simulink model "model"  (R2023b)
settings: Solver=VariableStepAuto  StartTime=0.0  StopTime=5  FixedStep=Tsi/10  RelTol=1e-4
undefined symbols (not defined in the file): B, B0, DiscIntNeverNeededParam, grtot, Hpp, Imax, In, Jm, Kdp_si, Ke, Ki_si, Kip_si, Kp_si, Kpp_si, Kppph_si, Kpppl_si, Kt, Kv, L, max_ppa_si, max_ppv_si, R, tauGp, Umax
libraries: simulink x10, slctrl_linear x1
(part 1 of 2)
settings Model: Creator=Giulio  LastModifiedBy=nicol
settings OptimizationCC: ReuseModelBlockBuffer=off
settings DebuggingCC: UnconnectedInputMsg=warning  UnconnectedOutputMsg=warning  UnconnectedLineMsg=warning
settings ModelReferenceCC: EnableRefExpFcnMdlSchedulingChecks=on

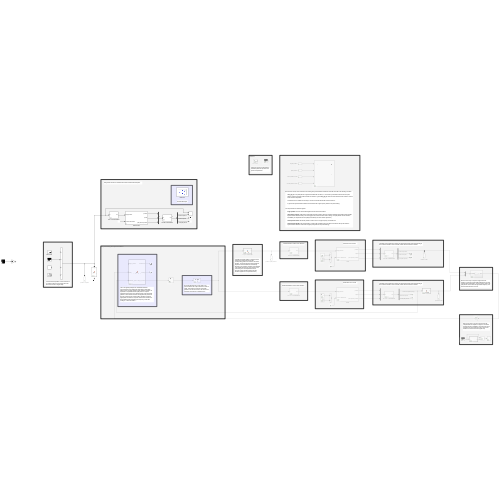
[thumbnail: Simulink's stored preview of the top-level diagram]
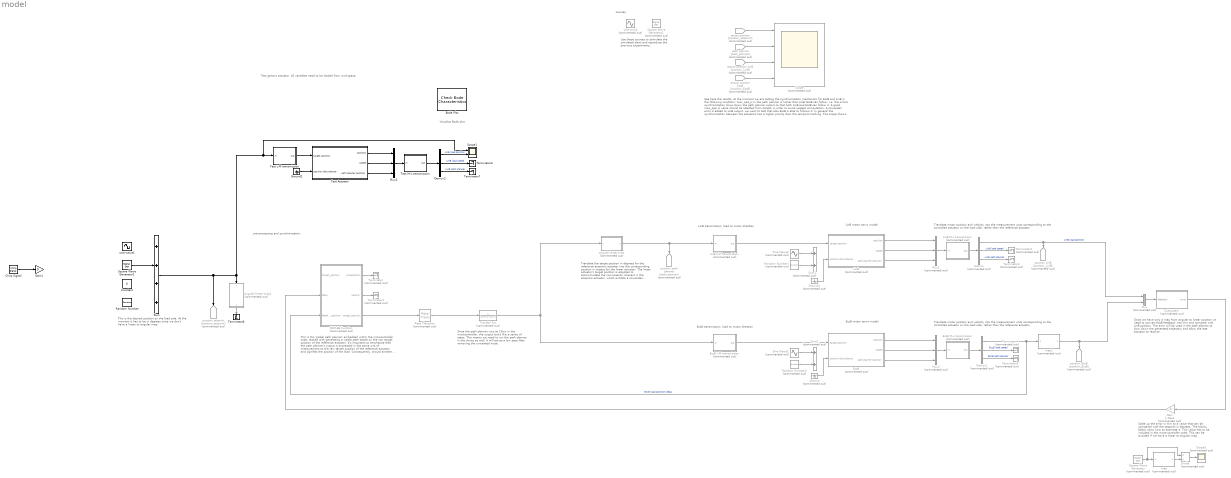
== system model ==
  note: This is the desired position on the load side. At the moment it has to be in degrees since we don't have a linear to angular map.
  note: This is the 'global path planner' embedded within the microcontroller code, tasked with generating a viable path based on the raw target position of the reference actuator. It's important to emphasize that the path planner's output is expressed in the same unit of measurement as the raw target position of the reference actuator and signifies the position of the load. Consequently, should another actuator be utilized, appropriate conversion is required. Note that the resolution of the generated path is limited by the frequency of the task running it, in this case 100Hz.
  note: sources
  note: Use these sources to stimulate the simulated plant and reproduce the previous experiments.
  note: pre-processing and synchronization
  note: Translate the target position in degrees for the reference eccentric actuator into the corresponding position in meters for the linear actuator. The linear actuator's target position is adjusted to accommodate the non-linearity inherent in the eccentric actuator, which exhibits a sinusoidal behavior due to the presence of a connecting rod. This adjustment ensures accurate synchronization between the two actuators (apart from unexpected blocks).
  note: Since the path planner runs at 10ms in the microcontroller, the output looks like a series of steps. This means we need to run the path planner in the drives as well. It will act as a low pass filter removing the unwanted noise.
  note: Translate motor position and velocity into the measurement units corresponding to the controlled actuator on the load side, rather than the reference actuator.
  note: Scale up the error in mm to a value that can be compared with the setpoint in degrees. The blocks below show how to estimate it. This value has to be included in the micro-controller code. This can be avoided if we have a linear to angular map.
  note: See here the results, at the moment we are testing the synchronization mechanism for EccB and LinB in the following condition:
      |
      | max_ppa_si in the path planner is higher that what EccB can follow, i.e. the online synchronization slows down the path planner output so that both LinB and EccB can follow it. A good max_ppa_si value should be selected from scratch in order to avoid useless computation.
      |
      | A sinusoidal error is added to LinB output, we want to test that also EccB is able to followo it.
      |
      | In general the synchronization between the actuators has a higher priority than the set-point tracking.
      |
      | The scope shows four different signals:
      |
      | target position : the raw commanded target that both drives should follow
      |
      | path planner position : path planner with double objective function (steer the actuators towards target position and maintain synchronization between them), note in the graph how, when the drives start to diverge, the path planner inverts direction immediately to compensate for thet (always bounded by the slow actuator dynamics).
      |
      | actual position LinB : LinB actual position to which we sum a high frequency sinusoidal error.
      |
      | actual position EccB : EccB actual position, it limits LinB acceleration at at the same time follows LinB (in this case the synchronization between motors has a higher priority than the set-point tracking).
  note: Since we have only a map from angular to linear position ve need to convert EccB feedback into mm and compare with LinB position. The error will be used in the path planner to slow down the generated trajectory and allow the late actuator to recover.
  note: LinB motor servo model
  note: EccB motor servo model
  note: LinB transmission: load to motor direction
  note: Translate motor position and velocity into the measurement units corresponding to the controlled actuator on the load side, rather than the reference actuator.
  note: EccB transmission: load to motor direction
  note: Visualize Bode plot
  note: Test generic actuator. All variables need to be loaded from workspace.
  Bode Plot : slctrl_linear/Check Bode  Characteristics  InstantiateOnLoad=on  SaveOperatingPoints=off  LinearizationIOs={'/Sum', 1, 'in', 'off', '';'/Demux2', 1, 'out', 'on', ''}  LinearizeAt=SnapshotTimes  SnapshotTimes=[0]  TriggerType=rising  SampleTime=auto  RateConversionMethod=zoh  PreWarpFreq=10  UseExactDelayModel=off  UseFullBlockNameLabels=off  UseBusSignalLabels=off  enabled=on  stopWhenAssertionFail=off  export=off  ViewDlgPos=[10 170 1856 825]  OpenViewOnLoad=off  LaunchViewOnOpen=on  FrequencyUnits=rad/s  MagnitudeUnits=dB  PhaseUnits=deg  TimeUnits=seconds  EnableUpperBound=off  UpperBoundFrequencies=[]  UpperBoundMagnitudes=[]  EnableLowerBound=off  LowerBoundFrequencies=[]  LowerBoundMagnitudes=[]
      settings: LibrarySourceBlock=slctrlblks/Linear Analysis Plots/Bode Plot  SaveToWorkspace=on  SaveName=sys
  Chirp Signal : simulink/Sources/Chirp Signal  f1=0.1  T=40  f2=5
  Constant : Constant  Value=0
  Demux : Demux  Commented=on  Outputs=3
  Demux1 : Demux  Commented=on  Outputs=3
  Demux2 : Demux  Outputs=3
  Divide : Product  Commented=on  Inputs=*/
  EccB : Subsystem  Commented=on  mask(Motor servo){Tsi=4e-5, Tsp=4e-4, Tspp=4e-4}
      mask DialogControl SamplingTimes Prompt: Sampling times
  EccB L-M transmission : Subsystem  Commented=on  mask(Transmission){gr_tot=2*pi*24.77/48, Direction=LOAD_TO_MOTOR}
      mask prompts: gr_tot "Total gear ratio"
      mask help: The total gear ratio represents the movement on motor side (in rad) correspondent to a displacement of one degree on load side.
      mask TypeOptions Direction: MOTOR_TO_LOAD | LOAD_TO_MOTOR
  EccB M-L transmission : Subsystem  Commented=on  mask(Transmission){gr_tot=2*pi*24.77/48, Direction=MOTOR_TO_LOAD}
      mask prompts: gr_tot "Total gear ratio"
      mask help: The total gear ratio represents the movement on motor side (in rad) correspondent to a displacement of one degree on load side.
      mask TypeOptions Direction: MOTOR_TO_LOAD | LOAD_TO_MOTOR
  Gain : Gain  Commented=on  Gain=1.48e4
  Gain1 : Gain  Gain=5
  Ground : Ground  Commented=on
  Ground1 : Ground  Commented=on
  Ground2 : Ground
  LinB : Subsystem  Commented=on  mask(Motor servo){Tsi=4e-5, Tsp=4e-4, Tspp=4e-4}
      mask DialogControl SamplingTimes Prompt: Sampling times
  LinB L-M transmission : Subsystem  Commented=on  mask(Transmission){gr_tot=1000*2*pi*174.72/48, Direction=LOAD_TO_MOTOR}
      mask prompts: gr_tot "Total gear ratio"
      mask help: The total gear ratio represents the movement on motor side (in rad) correspondent to a displacement of one meter on load side.
      mask TypeOptions Direction: MOTOR_TO_LOAD | LOAD_TO_MOTOR
  LinB M-L transmission : Subsystem  Commented=on  mask(Transmission){gr_tot=1000*2*pi*174.72/48, Direction=MOTOR_TO_LOAD}
      mask prompts: gr_tot "Total gear ratio"
      mask help: The total gear ratio represents the movement on motor side (in rad) correspondent to a displacement of one meter on load side.
      mask TypeOptions Direction: MOTOR_TO_LOAD | LOAD_TO_MOTOR
  MATLAB Function : MATLAB Function  Commented=on  TreatAsAtomicUnit=on  SystemSampleTime=Tspp  mask(High level path planner){Tspp=0.01, velocity_offset=1, Kppph_si=32.2971, Kpppl_si=3.2297, Hpp=12.5000, synch_to_target_ratio=1, max_ppv_si=155.6722, max_ppa_si=3.2297e+03}
      mask prompts: velocity_offset "Velocity hysteresis offset"; Kppph_si "Gain high limit"; Kpppl_si "Gain low limit"; Hpp "Exponential decay"; synch_to_target_ratio "Synch to target ratio"; max_ppv_si "Max velocity"; max_ppa_si "Max acceleration"
      mask help: Given a raw target trajectory, create a trajectory that all actuators are able to follow smoothly.
  Mux : Mux  Commented=on  Inputs=2
  Mux1 : Mux  Commented=on  Inputs=3
  Mux2 : Mux  Commented=on  Inputs=3
  Mux3 : Mux  Inputs=3
  Random Number : RandomNumber  Variance=1e-9  SampleTime=1e-3
  Random Number1 : RandomNumber  Commented=on  Variance=1e-6  SampleTime=1e-3
  Random Number2 : RandomNumber  Commented=on  Variance=1e-6  SampleTime=1e-3
  Rate Transition : RateTransition  Commented=on
  Scope : Scope  Commented=on  NumInputPorts=4
  Scope1 : Scope  NumInputPorts=2
  Scope3 : Scope  Commented=on
  Sine Wave1 : Sin  Commented=on  Amplitude=2e-4  Frequency=2*2*pi  SampleTime=0
  Sine Wave2 : Sin  Commented=on  Amplitude=2e-4  Frequency=2*2*pi  SampleTime=0
  Square Wave Generator : SignalGenerator  Commented=on  WaveForm=square
  Square Wave Generator1 : SignalGenerator  Commented=on  WaveForm=square  Amplitude=68.5  Frequency=0.5
  Square Wave Generator2 : SignalGenerator  WaveForm=square  Amplitude=-5  Frequency=0.4
  Subsystem : Subsystem  Commented=on
  Sum : Sum  Inputs=++++
  Sum1 : Sum  Commented=on
  Sum2 : Sum  Commented=on
  Terminator{,1..5} (6 alike) : Terminator  Commented=on
  Terminator6 : Terminator
  Terminator7 : Terminator
  Terminator8 : Terminator
  Test Actuator : Subsystem  mask(Motor servo){Tsi=4e-5, Tsp=4e-4, Tspp=4e-4}
      mask DialogControl SamplingTimes Prompt: Sampling times
  Test L-M transmission : Subsystem  mask(Transmission){gr_tot=grtot, Direction=LOAD_TO_MOTOR}
      mask prompts: gr_tot "Total gear ratio"
      mask help: The total gear ratio represents the movement on motor side (in rad) correspondent to a displacement of one meter on load side.
      mask TypeOptions Direction: MOTOR_TO_LOAD | LOAD_TO_MOTOR
  Test M-L transmission : Subsystem  mask(Transmission){gr_tot=grtot, Direction=MOTOR_TO_LOAD}
      mask prompts: gr_tot "Total gear ratio"
      mask help: The total gear ratio represents the movement on motor side (in rad) correspondent to a displacement of one meter on load side.
      mask TypeOptions Direction: MOTOR_TO_LOAD | LOAD_TO_MOTOR
  Transfer Fcn : TransferFcn  Commented=on  Denominator=[1/(2*pi*10) 1]
  actual position EccB : From  Commented=on  GotoTag=position_EccB
  actual position LinB : From  Commented=on  GotoTag=position_LinB
  angular-linear-map : MATLAB Function  Commented=on  TreatAsAtomicUnit=on
  angular-linear-map2 : MATLAB Function  Commented=on  TreatAsAtomicUnit=on
  map : MATLAB Function  Commented=on  TreatAsAtomicUnit=on
  map1 : MATLAB Function  Commented=on  TreatAsAtomicUnit=on
  path planner : From  Commented=on  GotoTag=path_planner
  position EccB : Goto  Commented=on  GotoTag=position_EccB
  position LinB : Goto  Commented=on  GotoTag=position_LinB
  position path planner : Goto  Commented=on  GotoTag=path_planner
  position setpoint : Goto  Commented=on  GotoTag=position_setpoint
  sine-wave : Sin  Commented=on  Amplitude=2.5e-3  Frequency=2*pi*2  SampleTime=0
  sine-wave1 : Sin  Amplitude=2.5e-3  Frequency=2*pi*17*3  SampleTime=0
  target position : From  Commented=on  GotoTag=position_setpoint
  wires:
  MATLAB Function/1(acceleration) -> Terminator/1
  MATLAB Function/2(velocity) -> Terminator1/1
  LinB M-L transmission/1(out) -> Demux/1
  Mux1/1 -> LinB M-L transmission/1(in)
  LinB/2(speed) -> Mux1/2
  LinB/1(position) -> Mux1/1
  LinB L-M transmission/1(out) -> LinB/1(target position)
  LinB/3(path planner position) -> Mux1/3
  Demux/2 -> Terminator2/1  "LinB load speed"
  Demux/3 -> Terminator3/1  "LinB path planner"
  EccB L-M transmission/1(out) -> EccB/1(target position)
  EccB/1(position) -> Mux2/1
  EccB/2(speed) -> Mux2/2
  EccB/3(path planner position) -> Mux2/3
  Mux2/1 -> EccB M-L transmission/1(in)
  EccB M-L transmission/1(out) -> Demux1/1
  Demux1/1 -> map1/1("x "), MATLAB Function/3(feedback_position)  "EccB load position [deg]"
  Demux1/2 -> Terminator4/1  "EccB load speed"
  Demux1/3 -> Terminator5/1  "EccB path planner"
  Mux/1 -> Subsystem/1(feedback)
  Transfer Fcn/1 -> EccB L-M transmission/1(in), angular-linear-map/1("x ")
  angular-linear-map/1(x) -> LinB L-M transmission/1(in), position path planner/1
  Subsystem/1(error) -> Gain/1
  map/1(x) -> Divide/2
  Square Wave Generator/1 -> Divide/1, map/1("x ")
  Divide/1 -> Scope3/1
  Gain/1 -> MATLAB Function/2(delay)
  Demux/1 -> position LinB/1, Mux/1  "LinB load position"
  actual position EccB/1 -> Scope/4
  actual position LinB/1 -> Scope/3
  target position/1 -> Scope/1
  path planner/1 -> Scope/2
  MATLAB Function/3(target_position) -> Rate Transition/1
  Rate Transition/1 -> Transfer Fcn/1
  map1/1(x) -> Mux/2, position EccB/1
  Sine Wave1/1 -> Sum1/1
  Random Number2/1 -> Sum1/2
  Random Number1/1 -> Sum2/2
  Sine Wave2/1 -> Sum2/1
  Ground/1 -> EccB/2(position disturbance)
  Ground1/1 -> LinB/2(position disturbance)
  Test L-M transmission/1(out) -> Test Actuator/1(target position)
  Test Actuator/3(path planner position) -> Mux3/3
  Test Actuator/2(speed) -> Mux3/2
  Mux3/1 -> Test M-L transmission/1(in)
  Test Actuator/1(position) -> Mux3/1
  Ground2/1 -> Test Actuator/2(position disturbance)
  Demux2/2 -> Terminator6/1  "LinB load speed"
  Demux2/3 -> Terminator7/1  "LinB path planner"
  Test M-L transmission/1(out) -> Demux2/1
  Demux2/1 -> Scope1/2  "LinB load position"
  Sum/1 -> position setpoint/1, Scope1/1, Test L-M transmission/1(in), angular-linear-map2/1("x ")
  angular-linear-map2/1(x) -> Terminator8/1
  Chirp Signal/1 -> Gain1/1
  Square Wave Generator2/1 -> Sum/2

== system model/EccB ==
  note: position control loop
  note: Employ a rate transmission block featuring a unity delay to replicate the time disparity between the sampling intervals of the position and current controllers.
  note: The position regulator takes multiple inputs, including the position setpoint, position feedback, and optionally, velocity and acceleration feedforward components. It then calculates and produces the necessary current signal to control the plant. This regulatory mechanism is implemented using a straightforward PID control scheme, complete with current saturation (limited to the motor's nominal current) and anti-windup provisions.
  note: motor path planner
  note: Drive internal path planner. It acts as low pass filter considering the physical limitation of the motor.
  target position : Inport
  position disturbance : Inport  Port=2
  Ground : Ground
  Rate Transition : RateTransition
  Sum : Sum
  Terminator{2..3,5..6} (4 alike) : Terminator
  current loop : Subsystem
  path planner : Subsystem  TreatAsAtomicUnit=on  SystemSampleTime=Tspp  mask(Drive internal path planner){Active=off, max_ppa_si=5.2360e+03, max_ppv_si=672.9990, Kppph_si=52.3599, Kpppl_si=5.2360, Hpp=12.5000}
      mask prompts: max_ppa_si "Max acceleration"; max_ppv_si "Max speed"; Kppph_si "High gain"; Kpppl_si "Low gain"; Hpp "Exponential"
      mask DialogControl ParameterGroupVar Prompt: Status
      mask DialogControl Container3 Prompt: Saturation
      mask DialogControl Container4 Prompt: Controller
  position regulator : Subsystem  TreatAsAtomicUnit=on  SystemSampleTime=Tsp  mask(Position PID controller){In=6.1800, Imax=27, Kpp_si=6, Kip_si=150, Kdp_si=0.06, FF_w_si=0, FF_a_si=0}
      mask prompts: In "Nominal current"; Imax "Max current"; Kpp_si "Proportional gain"; Kip_si "Integral gain"; Kdp_si "Derivative gain"; FF_w_si "Velocity feed forward gain"; FF_a_si "Acceleration feed forward gain"
      mask DialogControl Saturation Prompt: Saturation
      mask DialogControl Controller Prompt: Controller
  position : Outport
  speed : Outport  Port=2
  path planner position : Outport  Port=3
  wires:
  position regulator/1(current) -> Rate Transition/1
  current loop/1(position) -> Sum/1, position regulator/4(position_feedback)
  Rate Transition/1 -> current loop/1(current demand)
  current loop/4(voltage) -> Terminator5/1
  current loop/3(current) -> Terminator6/1
  path planner/2(motor speed) -> Terminator3/1
  path planner/1(motor acceleration) -> Terminator2/1
  Ground/1 -> position regulator/2(velocity feed forward), position regulator/1(acceleration feed forward)
  target position/1 -> path planner/1(motor_position)
  Sum/1 -> position/1
  path planner/3(motor position) -> path planner position/1, position regulator/3(position)
  current loop/2(velocity) -> speed/1
  position disturbance/1 -> Sum/2

== system model/EccB L-M transmission ==
  in : Inport
  Constant1 : Constant  Value=Direction
  Constant2 : Constant
  Equal : RelationalOperator  Operator===  OutDataTypeStr=boolean  RndMeth=Simplest  InputSameDT=off
  Switch : Switch  Criteria=u2 > Threshold  SaturateOnIntegerOverflow=off  InputSameDT=off
  gear ratio (L-M) : Gain  Gain=gr_tot
  inverse gear ratio (M-L) : Gain  Gain=1/gr_tot
  out : Outport
  wires:
  in/1 -> gear ratio (L-M)/1, inverse gear ratio (M-L)/1
  inverse gear ratio (M-L)/1 -> Switch/1
  gear ratio (L-M)/1 -> Switch/3
  Switch/1 -> out/1
  Constant1/1 -> Equal/1
  Equal/1 -> Switch/2
  Constant2/1 -> Equal/2

== system model/EccB M-L transmission ==
  in : Inport
  Constant1 : Constant  Value=Direction
  Constant2 : Constant
  Equal : RelationalOperator  Operator===  OutDataTypeStr=boolean  RndMeth=Simplest  InputSameDT=off
  Switch : Switch  Criteria=u2 > Threshold  SaturateOnIntegerOverflow=off  InputSameDT=off
  gear ratio (L-M) : Gain  Gain=gr_tot
  inverse gear ratio (M-L) : Gain  Gain=1/gr_tot
  out : Outport
  wires:
  in/1 -> gear ratio (L-M)/1, inverse gear ratio (M-L)/1
  inverse gear ratio (M-L)/1 -> Switch/1
  gear ratio (L-M)/1 -> Switch/3
  Switch/1 -> out/1
  Constant1/1 -> Equal/1
  Equal/1 -> Switch/2
  Constant2/1 -> Equal/2

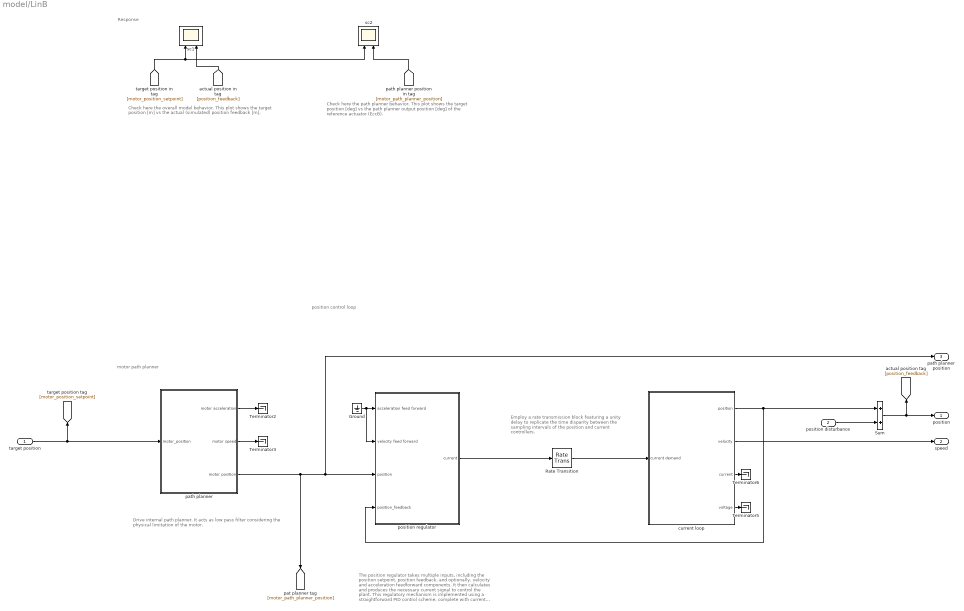
== system model/LinB ==
  note: position control loop
  note: Employ a rate transmission block featuring a unity delay to replicate the time disparity between the sampling intervals of the position and current controllers.
  note: The position regulator takes multiple inputs, including the position setpoint, position feedback, and optionally, velocity and acceleration feedforward components. It then calculates and produces the necessary current signal to control the plant. This regulatory mechanism is implemented using a straightforward PID control scheme, complete with current saturation (limited to the motor's nominal current) and anti-windup provisions.
  note: motor path planner
  note: Drive internal path planner. It acts as low pass filter considering the physical limitation of the motor.
  note: Response
  note: Check here the overall model behavior. This plot shows the target position [m] vs the actual (simulated) position feedback [m].
  note: Check here the path planner behavior. This plot shows the target position [deg] vs the path planner output position [deg] of the reference actuator (EccB).
  target position : Inport
  position disturbance : Inport  Port=2
  Ground : Ground
  Rate Transition : RateTransition
  Sum : Sum
  Terminator{2..3,5..6} (4 alike) : Terminator
  current loop : Subsystem
  path planner : Subsystem  TreatAsAtomicUnit=on  SystemSampleTime=Tspp  mask(Drive internal path planner){Active=off, max_ppa_si=2.0944e+03, max_ppv_si=656.2438, Kppph_si=20.9440, Kpppl_si=2.0944, Hpp=12.5000}
      mask prompts: max_ppa_si "Max acceleration"; max_ppv_si "Max speed"; Kppph_si "High gain"; Kpppl_si "Low gain"; Hpp "Exponential"
      mask DialogControl ParameterGroupVar Prompt: Status
      mask DialogControl Container3 Prompt: Saturation
      mask DialogControl Container4 Prompt: Controller
  position regulator : Subsystem  TreatAsAtomicUnit=on  SystemSampleTime=Tsp  mask(Position PID controller){In=4.2700, Imax=22, Kpp_si=2.5, Kip_si=50, Kdp_si=0.025, FF_w_si=0, FF_a_si=0}
      mask prompts: In "Nominal current"; Imax "Max current"; Kpp_si "Proportional gain"; Kip_si "Integral gain"; Kdp_si "Derivative gain"; FF_w_si "Velocity feed forward gain"; FF_a_si "Acceleration feed forward gain"
      mask DialogControl Saturation Prompt: Saturation
      mask DialogControl Controller Prompt: Controller
  sc1 : Scope  NumInputPorts=2
  sc2 : Scope  NumInputPorts=2
  position : Outport
  speed : Outport  Port=2
  path planner position : Outport  Port=3
  wires:
  path planner/3(motor position) -> path planner position/1, position regulator/3(position), [motor_path_planner_position]
  position regulator/1(current) -> Rate Transition/1
  current loop/1(position) -> Sum/1, position regulator/4(position_feedback)
  Rate Transition/1 -> current loop/1(current demand)
  current loop/4(voltage) -> Terminator5/1
  current loop/3(current) -> Terminator6/1
  path planner/2(motor speed) -> Terminator3/1
  path planner/1(motor acceleration) -> Terminator2/1
  Ground/1 -> position regulator/2(velocity feed forward), position regulator/1(acceleration feed forward)
  target position/1 -> [motor_position_setpoint], path planner/1(motor_position)
  current loop/2(velocity) -> speed/1
  [motor_position_setpoint] -> sc2/1, sc1/1
  [position_feedback] -> sc1/2
  [motor_path_planner_position] -> sc2/2
  position disturbance/1 -> Sum/2
  Sum/1 -> [position_feedback], position/1

== system model/LinB L-M transmission ==
  in : Inport
  Constant1 : Constant  Value=Direction
  Constant2 : Constant
  Equal : RelationalOperator  Operator===  OutDataTypeStr=boolean  RndMeth=Simplest  InputSameDT=off
  Switch : Switch  Criteria=u2 > Threshold  SaturateOnIntegerOverflow=off  InputSameDT=off
  gear ratio (L-M) : Gain  Gain=gr_tot
  inverse gear ratio (M-L) : Gain  Gain=1/gr_tot
  out : Outport
  wires:
  in/1 -> gear ratio (L-M)/1, inverse gear ratio (M-L)/1
  inverse gear ratio (M-L)/1 -> Switch/1
  gear ratio (L-M)/1 -> Switch/3
  Switch/1 -> out/1
  Constant1/1 -> Equal/1
  Equal/1 -> Switch/2
  Constant2/1 -> Equal/2

== system model/LinB M-L transmission ==
  in : Inport
  Constant1 : Constant  Value=Direction
  Constant2 : Constant
  Equal : RelationalOperator  Operator===  OutDataTypeStr=boolean  RndMeth=Simplest  InputSameDT=off
  Switch : Switch  Criteria=u2 > Threshold  SaturateOnIntegerOverflow=off  InputSameDT=off
  gear ratio (L-M) : Gain  Gain=gr_tot
  inverse gear ratio (M-L) : Gain  Gain=1/gr_tot
  out : Outport
  wires:
  in/1 -> gear ratio (L-M)/1, inverse gear ratio (M-L)/1
  inverse gear ratio (M-L)/1 -> Switch/1
  gear ratio (L-M)/1 -> Switch/3
  Switch/1 -> out/1
  Constant1/1 -> Equal/1
  Equal/1 -> Switch/2
  Constant2/1 -> Equal/2

== system model/Subsystem ==
  feedback : Inport
  MinMax : MinMax
  MinMax1 : MinMax  Function=max
  Selector : Selector  InputPortWidth=3  IndexOptions=Index vector (dialog)  Indices=1  OutputSizes=1
  Sum : Sum  Inputs=+-
  error : Outport
  wires:
  feedback/1 -> MinMax/1, MinMax1/1
  MinMax1/1 -> Sum/1
  MinMax/1 -> Sum/2
  Sum/1 -> Selector/1
  Selector/1 -> error/1

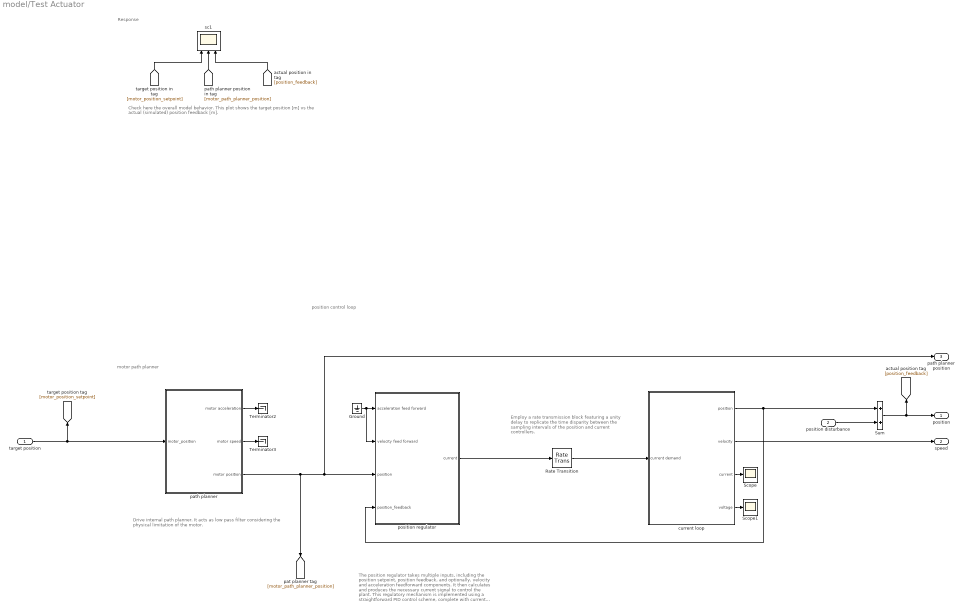
== system model/Test Actuator ==
  note: position control loop
  note: Employ a rate transmission block featuring a unity delay to replicate the time disparity between the sampling intervals of the position and current controllers.
  note: The position regulator takes multiple inputs, including the position setpoint, position feedback, and optionally, velocity and acceleration feedforward components. It then calculates and produces the necessary current signal to control the plant. This regulatory mechanism is implemented using a straightforward PID control scheme, complete with current saturation (limited to the motor's nominal current) and anti-windup provisions.
  note: motor path planner
  note: Drive internal path planner. It acts as low pass filter considering the physical limitation of the motor.
  note: Response
  note: Check here the overall model behavior. This plot shows the target position [m] vs the actual (simulated) position feedback [m].
  target position : Inport
  position disturbance : Inport  Port=2
  Ground : Ground
  Rate Transition : RateTransition
  Scope : Scope
  Scope1 : Scope
  Sum : Sum
  Terminator2 : Terminator
  Terminator3 : Terminator
  current loop : Subsystem
  path planner : Subsystem  TreatAsAtomicUnit=on  SystemSampleTime=Tspp  mask(Drive internal path planner){Active=off, max_ppa_si=max_ppa_si, max_ppv_si=max_ppv_si, Kppph_si=Kppph_si, Kpppl_si=Kpppl_si, Hpp=Hpp}
      mask prompts: max_ppa_si "Max acceleration"; max_ppv_si "Max speed"; Kppph_si "High gain"; Kpppl_si "Low gain"; Hpp "Exponential"
      mask DialogControl ParameterGroupVar Prompt: Status
      mask DialogControl Container3 Prompt: Saturation
      mask DialogControl Container4 Prompt: Controller
  position regulator : Subsystem  TreatAsAtomicUnit=on  SystemSampleTime=Tsp  mask(Position PID controller){In=In, Imax=Imax, Kpp_si=Kpp_si, Kip_si=Kip_si, Kdp_si=Kdp_si, FF_w_si=0, FF_a_si=0}
      mask prompts: In "Nominal current"; Imax "Max current"; Kpp_si "Proportional gain"; Kip_si "Integral gain"; Kdp_si "Derivative gain"; FF_w_si "Velocity feed forward gain"; FF_a_si "Acceleration feed forward gain"
      mask DialogControl Saturation Prompt: Saturation
      mask DialogControl Controller Prompt: Controller
  sc1 : Scope  NumInputPorts=3
  position : Outport
  speed : Outport  Port=2
  path planner position : Outport  Port=3
  wires:
  position regulator/1(current) -> Rate Transition/1
  current loop/1(position) -> Sum/1, position regulator/4(position_feedback)
  Rate Transition/1 -> current loop/1(current demand)
  current loop/4(voltage) -> Scope1/1
  current loop/3(current) -> Scope/1
  path planner/2(motor speed) -> Terminator3/1
  path planner/1(motor acceleration) -> Terminator2/1
  Ground/1 -> position regulator/2(velocity feed forward), position regulator/1(acceleration feed forward)
  target position/1 -> [motor_position_setpoint], path planner/1(motor_position)
  current loop/2(velocity) -> speed/1
  [motor_position_setpoint] -> sc1/1
  position disturbance/1 -> Sum/2
  Sum/1 -> [position_feedback], position/1
  [position_feedback] -> sc1/3
  [motor_path_planner_position] -> sc1/2
  path planner/3(motor position) -> [motor_path_planner_position], path planner position/1, position regulator/3(position)

== system model/Test L-M transmission ==
  in : Inport
  Constant1 : Constant  Value=Direction
  Constant2 : Constant
  Equal : RelationalOperator  Operator===  OutDataTypeStr=boolean  RndMeth=Simplest  InputSameDT=off
  Switch : Switch  Criteria=u2 > Threshold  SaturateOnIntegerOverflow=off  InputSameDT=off
  gear ratio (L-M) : Gain  Gain=gr_tot
  inverse gear ratio (M-L) : Gain  Gain=1/gr_tot
  out : Outport
  wires:
  in/1 -> gear ratio (L-M)/1, inverse gear ratio (M-L)/1
  inverse gear ratio (M-L)/1 -> Switch/1
  gear ratio (L-M)/1 -> Switch/3
  Switch/1 -> out/1
  Constant1/1 -> Equal/1
  Equal/1 -> Switch/2
  Constant2/1 -> Equal/2

== system model/Test M-L transmission ==
  in : Inport
  Constant1 : Constant  Value=Direction
  Constant2 : Constant
  Equal : RelationalOperator  Operator===  OutDataTypeStr=boolean  RndMeth=Simplest  InputSameDT=off
  Switch : Switch  Criteria=u2 > Threshold  SaturateOnIntegerOverflow=off  InputSameDT=off
  gear ratio (L-M) : Gain  Gain=gr_tot
  inverse gear ratio (M-L) : Gain  Gain=1/gr_tot
  out : Outport
  wires:
  in/1 -> gear ratio (L-M)/1, inverse gear ratio (M-L)/1
  inverse gear ratio (M-L)/1 -> Switch/1
  gear ratio (L-M)/1 -> Switch/3
  Switch/1 -> out/1
  Constant1/1 -> Equal/1
  Equal/1 -> Switch/2
  Constant2/1 -> Equal/2

== system model/EccB/current loop ==
  note: The current regulator receives input in the form of the desired current and current feedback from the plant, subsequently applying the requisite voltage to drive the BLDC motor. This regulation is achieved through the implementation of a PI controller, which incorporates voltage saturation (limited to the motor's nominal voltage) and anti-windup mechanisms.
  note: Second order BLDC motor model takes the desired voltage and the load inertia (adjusted for the motor side using the gear ratio) as inputs and produces outputs for position, velocity, and current. It serves as a basic representation solely for simulation purposes, with the potential for more detailed and improved implementation in future iterations.
  note: Here the Power supply could be modelled. Pay attention to this because on the car the voltage supply is not always constant and it has to be taken into account.
  note: First order BLDC motor model used to check that the parameter estimation is not to bad. Can be used as observer + Luenberg in the future if needed.
  current demand : Inport
  Scope : Scope  NumInputPorts=2
  Scope1 : Scope  NumInputPorts=2
  current regulator : Subsystem  TreatAsAtomicUnit=on  SystemSampleTime=Tsi  mask(Current PI controller){Umax=48, Un=36, Kp_si=0.9689, Ki_si=603.1858}
      mask prompts: Umax "Max voltage"; Un "Nominal voltage"; Kp_si "Proportional gain"; Ki_si "Integral gain"
      mask DialogControl Saturation Prompt: Saturation
      mask DialogControl Controller Prompt: Controller
  first order plant : Subsystem  mask(Motor first order plant){tauM=5.4400e-04, Kv=14.1372}
      mask prompts: tauM "Mechanical time constant"; Kv "Velocity constant"
      mask DialogControl Motor Prompt: Motor
  power supply : Subsystem
  second order plant : Subsystem  mask(Motor second order model){Ke=0.0706, R=0.16, L=2.5700e-04, Kt=0.0706, Jm=1.8290e-05, B=7.0915e-05, B0=0}
      mask prompts: Ke "Electrical constant"; R "Resistance"; L "Inductance"; Kt "Torque constant"; Jm "Motor inertia"; B "Viscous friction"; B0 "Static friction"
      mask DialogControl electrical Prompt: Electrical
      mask DialogControl Mechanical Prompt: Mechanical
  position : Outport
  velocity : Outport  Port=2
  current : Outport  Port=3
  voltage : Outport  Port=4
  wires:
  second order plant/2(velocity) -> Scope1/1, velocity/1
  current demand/1 -> current regulator/1(current)
  second order plant/1(position) -> Scope/1, position/1
  second order plant/3(current) -> current regulator/2(current_feedback), current/1
  power supply/1(voltage) -> second order plant/1(voltage), voltage/1
  current regulator/1(voltage) -> first order plant/1(voltage), power supply/1(voltage setpoint)
  first order plant/1(position) -> Scope/2
  first order plant/2(velocity) -> Scope1/2

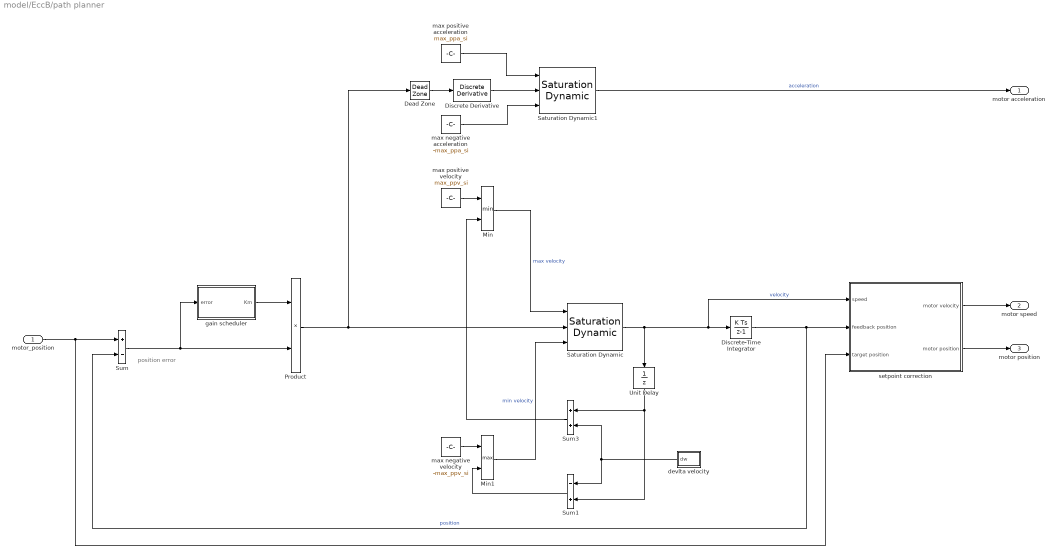
== system model/EccB/path planner ==
  note: position error
  motor_position : Inport
  Dead Zone : DeadZone  LowerValue=-0.01  UpperValue=0.01
  Discrete Derivative : simulink/Discrete/Discrete Derivative  gainval=1.0  ICPrevScaledInput=0.0  OutMin=[]  OutMax=[]  OutDataType=fixdt(1, 16)  OutScaling=2^-10  DoSatur=off
  Discrete-Time Integrator : DiscreteIntegrator  SampleTime=-1  ICPrevOutput=DiscIntNeverNeededParam  ICPrevScaledInput=DiscIntNeverNeededParam
  Min : MinMax  Inputs=2
  Min1 : MinMax  Function=max  Inputs=2
  Product : Product
  Saturation Dynamic : simulink/Discontinuities/Saturation Dynamic  OutMin=[]  OutMax=[]  OutDataTypeStr=Inherit: Same as second input  OutDataType=fixdt(1, 16)  OutScaling=2^-10  DoSatur=off
  Saturation Dynamic1 : simulink/Discontinuities/Saturation Dynamic  OutMin=[]  OutMax=[]  OutDataTypeStr=Inherit: Same as second input  OutDataType=fixdt(1, 16)  OutScaling=2^-10  DoSatur=off
  Sum : Sum  Inputs=+-
  Sum1 : Sum  Inputs=-+
  Sum3 : Sum
  Unit Delay : UnitDelay  SampleTime=-1  HasFrameUpgradeWarning=on
  devlta velocity : Subsystem
  gain scheduler : Subsystem
  max negative acceleration : Constant  Value=-max_ppa_si
  max negative velocity : Constant  Value=-max_ppv_si
  max positive acceleration : Constant  Value=max_ppa_si
  max positive velocity : Constant  Value=max_ppv_si
  setpoint correction : Subsystem
  motor acceleration : Outport
  motor speed : Outport  Port=2
  motor position : Outport  Port=3
  wires:
  Sum/1 -> gain scheduler/1(error), Product/2
  max positive velocity/1 -> Min/1
  Saturation Dynamic/1 -> setpoint correction/1(speed), Discrete-Time Integrator/1, Unit Delay/1  "velocity"
  devlta velocity/1(dw) -> Sum1/1, Sum3/2
  Sum3/1 -> Min/2
  max negative velocity/1 -> Min1/1
  Sum1/1 -> Min1/2
  Min1/1 -> Saturation Dynamic/3  "min velocity"
  Min/1 -> Saturation Dynamic/1  "max velocity"
  Discrete-Time Integrator/1 -> setpoint correction/2(feedback position), Sum/2  "position"
  Unit Delay/1 -> Sum1/2, Sum3/1
  max positive acceleration/1 -> Saturation Dynamic1/1
  max negative acceleration/1 -> Saturation Dynamic1/3
  Saturation Dynamic1/1 -> motor acceleration/1  "acceleration"
  Discrete Derivative/1 -> Saturation Dynamic1/2
  Dead Zone/1 -> Discrete Derivative/1
  setpoint correction/1(motor velocity) -> motor speed/1
  gain scheduler/1(Km) -> Product/1
  motor_position/1 -> setpoint correction/3(target position), Sum/1
  setpoint correction/2(motor position) -> motor position/1
  Product/1 -> Dead Zone/1, Saturation Dynamic/2

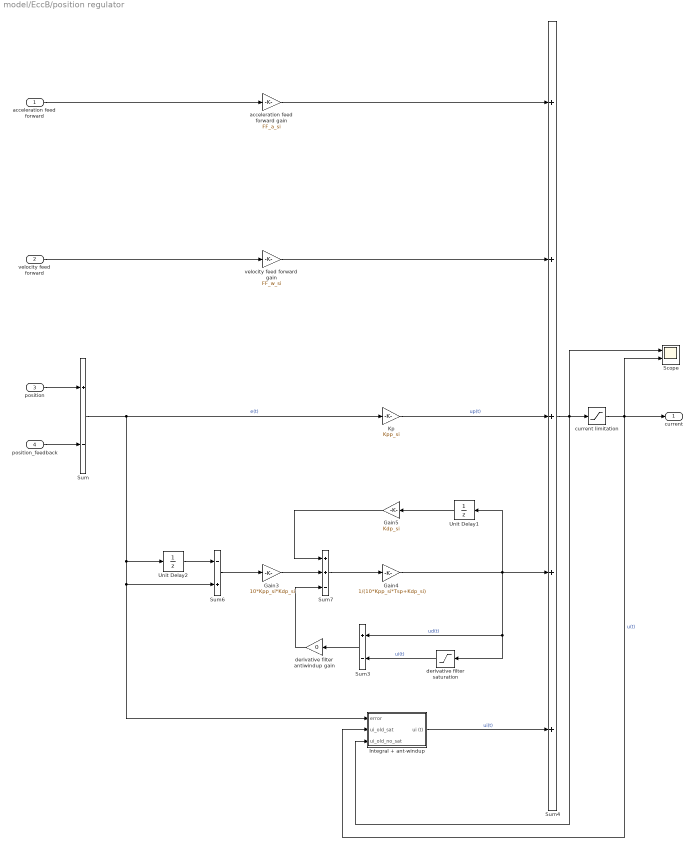
== system model/EccB/position regulator ==
  acceleration feed forward : Inport
  velocity feed forward : Inport  Port=2
  position : Inport  Port=3
  position_feedback : Inport  Port=4
  Gain3 : Gain  Gain=10*Kpp_si*Kdp_si
  Gain4 : Gain  Gain=1/(10*Kpp_si*Tsp+Kdp_si)
  Gain5 : Gain  Gain=Kdp_si
  Integral + ant-windup : Subsystem
  Kp : Gain  Gain=Kpp_si
  Scope : Scope  NumInputPorts=2
  Sum : Sum  Inputs=+-
  Sum3 : Sum  Inputs=+-
  Sum4 : Sum  Inputs=+++++
  Sum6 : Sum  Inputs=-+
  Sum7 : Sum  Inputs=++-
  Unit Delay1 : UnitDelay  SampleTime=-1  HasFrameUpgradeWarning=on
  Unit Delay2 : UnitDelay  SampleTime=-1  HasFrameUpgradeWarning=on
  acceleration feed forward gain : Gain  Gain=FF_a_si
  current limitation : Saturate  UpperLimit=Imax  LowerLimit=-Imax
  derivative filter antiwindup gain : Gain  Gain=0
  derivative filter saturation : Saturate  UpperLimit=Imax/2  LowerLimit=-Imax/2
  velocity feed forward gain : Gain  Gain=FF_w_si
  current : Outport
  wires:
  acceleration feed forward gain/1 -> Sum4/1
  acceleration feed forward/1 -> acceleration feed forward gain/1
  velocity feed forward gain/1 -> Sum4/2
  velocity feed forward/1 -> velocity feed forward gain/1
  Sum7/1 -> Gain4/1
  current limitation/1 -> current/1, Scope/2, Integral + ant-windup/2(ui_old_sat)  "u(t)"
  Unit Delay2/1 -> Sum6/1
  Sum6/1 -> Gain3/1
  Unit Delay1/1 -> Gain5/1
  Kp/1 -> Sum4/3  "up(t)"
  Sum/1 -> Kp/1, Integral + ant-windup/1(error), Sum6/2, Unit Delay2/1  "e(t)"
  Gain3/1 -> Sum7/2
  Gain5/1 -> Sum7/1
  Gain4/1 -> Sum4/4, derivative filter saturation/1, Sum3/1, Unit Delay1/1  "ud(t)"
  Sum3/1 -> derivative filter antiwindup gain/1
  derivative filter saturation/1 -> Sum3/2  "ui(t)"
  derivative filter antiwindup gain/1 -> Sum7/3
  Integral + ant-windup/1(ui (t)) -> Sum4/5  "ui(t)"
  Sum4/1 -> Scope/1, current limitation/1, Integral + ant-windup/3(ui_old_no_sat)
  position/1 -> Sum/1
  position_feedback/1 -> Sum/2

== system model/LinB/current loop ==
  note: The current regulator receives input in the form of the desired current and current feedback from the plant, subsequently applying the requisite voltage to drive the BLDC motor. This regulation is achieved through the implementation of a PI controller, which incorporates voltage saturation (limited to the motor's nominal voltage) and anti-windup mechanisms.
  note: Second order BLDC motor model takes the desired voltage and the load inertia (adjusted for the motor side using the gear ratio) as inputs and produces outputs for position, velocity, and current. It serves as a basic representation solely for simulation purposes, with the potential for more detailed and improved implementation in future iterations.
  note: Here the Power supply could be modelled. Pay attention to this because on the car the voltage supply is not always constant and it has to be taken into account.
  note: First order BLDC motor model used to check that the parameter estimation is not to bad. Can be used as observer + Luenberg in the future if needed.
  current demand : Inport
  Scope : Scope  NumInputPorts=2
  Scope1 : Scope  NumInputPorts=2
  current regulator : Subsystem  TreatAsAtomicUnit=on  SystemSampleTime=Tsi  mask(Current PI controller){Umax=48, Un=36, Kp_si=1.9302, Ki_si=1.9943e+03}
      mask prompts: Umax "Max voltage"; Un "Nominal voltage"; Kp_si "Proportional gain"; Ki_si "Integral gain"
      mask DialogControl Saturation Prompt: Saturation
      mask DialogControl Controller Prompt: Controller
  first order plant : Subsystem  mask(Motor first order plant){tauM=7.7800e-04, Kv=13.7183}
      mask prompts: tauM "Mechanical time constant"; Kv "Velocity constant"
      mask DialogControl Motor Prompt: Motor
  power supply : Subsystem
  second order plant : Subsystem  mask(Motor second order model){Ke=0.0728, R=0.5290, L=5.1200e-04, Kt=0.0728, Jm=9.2000e-06, B=3.6682e-05, B0=0}
      mask prompts: Ke "Electrical constant"; R "Resistance"; L "Inductance"; Kt "Torque constant"; Jm "Motor inertia"; B "Viscous friction"; B0 "Static friction"
      mask DialogControl electrical Prompt: Electrical
      mask DialogControl Mechanical Prompt: Mechanical
  position : Outport
  velocity : Outport  Port=2
  current : Outport  Port=3
  voltage : Outport  Port=4
  wires:
  second order plant/2(velocity) -> Scope1/1, velocity/1
  current demand/1 -> current regulator/1(current)
  second order plant/1(position) -> Scope/1, position/1
  second order plant/3(current) -> current regulator/2(current_feedback), current/1
  power supply/1(voltage) -> second order plant/1(voltage), voltage/1
  current regulator/1(voltage) -> first order plant/1(voltage), power supply/1(voltage setpoint)
  first order plant/1(position) -> Scope/2
  first order plant/2(velocity) -> Scope1/2

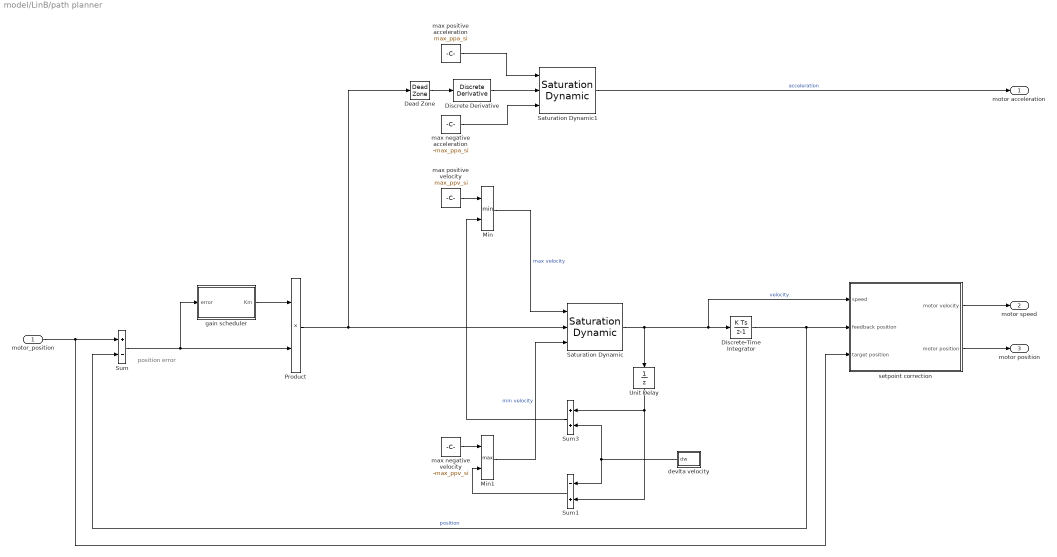
== system model/LinB/path planner ==
  note: position error
  motor_position : Inport
  Dead Zone : DeadZone  LowerValue=-0.01  UpperValue=0.01
  Discrete Derivative : simulink/Discrete/Discrete Derivative  gainval=1.0  ICPrevScaledInput=0.0  OutMin=[]  OutMax=[]  OutDataType=fixdt(1, 16)  OutScaling=2^-10  DoSatur=off
  Discrete-Time Integrator : DiscreteIntegrator  SampleTime=Tspp  ICPrevOutput=DiscIntNeverNeededParam  ICPrevScaledInput=DiscIntNeverNeededParam
  Min : MinMax  Inputs=2
  Min1 : MinMax  Function=max  Inputs=2
  Product : Product
  Saturation Dynamic : simulink/Discontinuities/Saturation Dynamic  OutMin=[]  OutMax=[]  OutDataTypeStr=Inherit: Same as second input  OutDataType=fixdt(1, 16)  OutScaling=2^-10  DoSatur=off
  Saturation Dynamic1 : simulink/Discontinuities/Saturation Dynamic  OutMin=[]  OutMax=[]  OutDataTypeStr=Inherit: Same as second input  OutDataType=fixdt(1, 16)  OutScaling=2^-10  DoSatur=off
  Sum : Sum  Inputs=+-
  Sum1 : Sum  Inputs=-+
  Sum3 : Sum
  Unit Delay : UnitDelay  SampleTime=-1  HasFrameUpgradeWarning=on
  devlta velocity : Subsystem
  gain scheduler : Subsystem
  max negative acceleration : Constant  Value=-max_ppa_si
  max negative velocity : Constant  Value=-max_ppv_si
  max positive acceleration : Constant  Value=max_ppa_si
  max positive velocity : Constant  Value=max_ppv_si
  setpoint correction : Subsystem
  motor acceleration : Outport
  motor speed : Outport  Port=2
  motor position : Outport  Port=3
  wires:
  Sum/1 -> gain scheduler/1(error), Product/2
  max positive velocity/1 -> Min/1
  Saturation Dynamic/1 -> setpoint correction/1(speed), Discrete-Time Integrator/1, Unit Delay/1  "velocity"
  devlta velocity/1(dw) -> Sum1/1, Sum3/2
  Sum3/1 -> Min/2
  max negative velocity/1 -> Min1/1
  Sum1/1 -> Min1/2
  Min1/1 -> Saturation Dynamic/3  "min velocity"
  Min/1 -> Saturation Dynamic/1  "max velocity"
  Discrete-Time Integrator/1 -> setpoint correction/2(feedback position), Sum/2  "position"
  Unit Delay/1 -> Sum1/2, Sum3/1
  max positive acceleration/1 -> Saturation Dynamic1/1
  max negative acceleration/1 -> Saturation Dynamic1/3
  Saturation Dynamic1/1 -> motor acceleration/1  "acceleration"
  Discrete Derivative/1 -> Saturation Dynamic1/2
  Dead Zone/1 -> Discrete Derivative/1
  setpoint correction/1(motor velocity) -> motor speed/1
  gain scheduler/1(Km) -> Product/1
  motor_position/1 -> setpoint correction/3(target position), Sum/1
  setpoint correction/2(motor position) -> motor position/1
  Product/1 -> Dead Zone/1, Saturation Dynamic/2

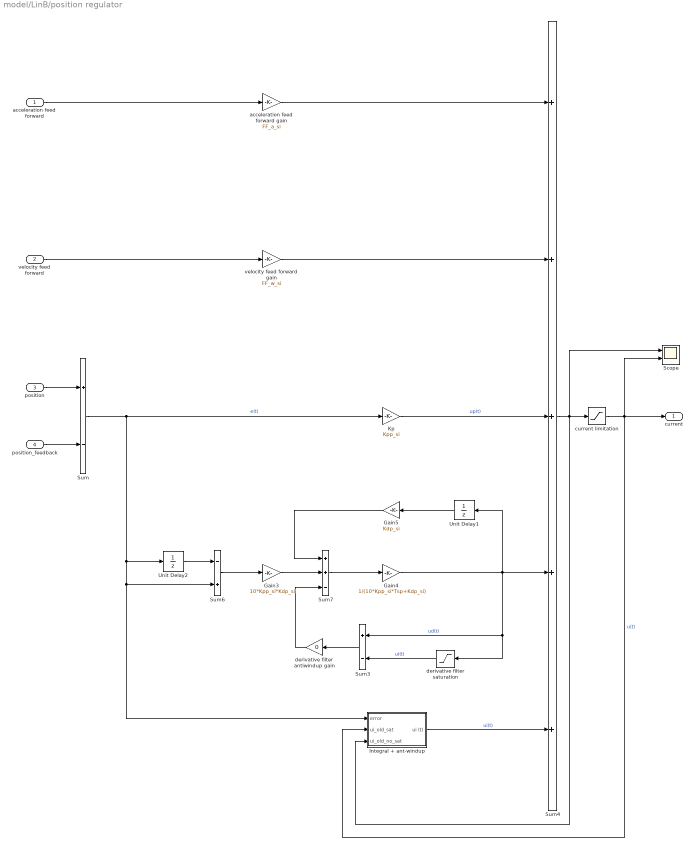
== system model/LinB/position regulator ==
  acceleration feed forward : Inport
  velocity feed forward : Inport  Port=2
  position : Inport  Port=3
  position_feedback : Inport  Port=4
  Gain3 : Gain  Gain=10*Kpp_si*Kdp_si
  Gain4 : Gain  Gain=1/(10*Kpp_si*Tsp+Kdp_si)
  Gain5 : Gain  Gain=Kdp_si
  Integral + ant-windup : Subsystem
  Kp : Gain  Gain=Kpp_si
  Scope : Scope  NumInputPorts=2
  Sum : Sum  Inputs=+-
  Sum3 : Sum  Inputs=+-
  Sum4 : Sum  Inputs=+++++
  Sum6 : Sum  Inputs=-+
  Sum7 : Sum  Inputs=++-
  Unit Delay1 : UnitDelay  SampleTime=-1  HasFrameUpgradeWarning=on
  Unit Delay2 : UnitDelay  SampleTime=-1  HasFrameUpgradeWarning=on
  acceleration feed forward gain : Gain  Gain=FF_a_si
  current limitation : Saturate  UpperLimit=Imax  LowerLimit=-Imax
  derivative filter antiwindup gain : Gain  Gain=0
  derivative filter saturation : Saturate  UpperLimit=Imax/2  LowerLimit=-Imax/2
  velocity feed forward gain : Gain  Gain=FF_w_si
  current : Outport
  wires:
  acceleration feed forward gain/1 -> Sum4/1
  acceleration feed forward/1 -> acceleration feed forward gain/1
  velocity feed forward gain/1 -> Sum4/2
  velocity feed forward/1 -> velocity feed forward gain/1
  Sum7/1 -> Gain4/1
  current limitation/1 -> current/1, Scope/2, Integral + ant-windup/2(ui_old_sat)  "u(t)"
  Unit Delay2/1 -> Sum6/1
  Sum6/1 -> Gain3/1
  Unit Delay1/1 -> Gain5/1
  Kp/1 -> Sum4/3  "up(t)"
  Sum/1 -> Kp/1, Integral + ant-windup/1(error), Sum6/2, Unit Delay2/1  "e(t)"
  Gain3/1 -> Sum7/2
  Gain5/1 -> Sum7/1
  Gain4/1 -> Sum4/4, derivative filter saturation/1, Sum3/1, Unit Delay1/1  "ud(t)"
  Sum3/1 -> derivative filter antiwindup gain/1
  derivative filter saturation/1 -> Sum3/2  "ui(t)"
  derivative filter antiwindup gain/1 -> Sum7/3
  Integral + ant-windup/1(ui (t)) -> Sum4/5  "ui(t)"
  Sum4/1 -> Scope/1, current limitation/1, Integral + ant-windup/3(ui_old_no_sat)
  position/1 -> Sum/1
  position_feedback/1 -> Sum/2

== system model/Test Actuator/current loop ==
  note: The current regulator receives input in the form of the desired current and current feedback from the plant, subsequently applying the requisite voltage to drive the BLDC motor. This regulation is achieved through the implementation of a PI controller, which incorporates voltage saturation (limited to the motor's nominal voltage) and anti-windup mechanisms.
  note: Second order BLDC motor model takes the desired voltage and the load inertia (adjusted for the motor side using the gear ratio) as inputs and produces outputs for position, velocity, and current. It serves as a basic representation solely for simulation purposes, with the potential for more detailed and improved implementation in future iterations.
  note: Here the Power supply could be modelled. Pay attention to this because on the car the voltage supply is not always constant and it has to be taken into account.
  note: First order BLDC motor model used to check that the parameter estimation is not to bad. Can be used as observer + Luenberg in the future if needed.
  current demand : Inport
  Scope : Scope  NumInputPorts=2
  Scope1 : Scope  NumInputPorts=2
  current regulator : Subsystem  TreatAsAtomicUnit=on  SystemSampleTime=Tsi  mask(Current PI controller){Umax=Umax, Un=Umax, Kp_si=Kp_si, Ki_si=Ki_si}
      mask prompts: Umax "Max voltage"; Un "Nominal voltage"; Kp_si "Proportional gain"; Ki_si "Integral gain"
      mask DialogControl Saturation Prompt: Saturation
      mask DialogControl Controller Prompt: Controller
  first order plant : Subsystem  mask(Motor first order plant){tauM=tauGp, Kv=Kv}
      mask prompts: tauM "Mechanical time constant"; Kv "Velocity constant"
      mask DialogControl Motor Prompt: Motor
  power supply : Subsystem
  second order plant : Subsystem  mask(Motor second order model){Ke=Ke, R=R, L=L, Kt=Kt, Jm=Jm, B=B, B0=B0}
      mask prompts: Ke "Electrical constant"; R "Resistance"; L "Inductance"; Kt "Torque constant"; Jm "Motor inertia"; B "Viscous friction"; B0 "Static friction"
      mask DialogControl electrical Prompt: Electrical
      mask DialogControl Mechanical Prompt: Mechanical
  position : Outport
  velocity : Outport  Port=2
  current : Outport  Port=3
  voltage : Outport  Port=4
  wires:
  second order plant/2(velocity) -> Scope1/1, velocity/1
  current demand/1 -> current regulator/1(current)
  second order plant/1(position) -> Scope/1, position/1
  second order plant/3(current) -> current regulator/2(current_feedback), current/1
  power supply/1(voltage) -> second order plant/1(voltage), voltage/1
  current regulator/1(voltage) -> first order plant/1(voltage), power supply/1(voltage setpoint)
  first order plant/1(position) -> Scope/2
  first order plant/2(velocity) -> Scope1/2

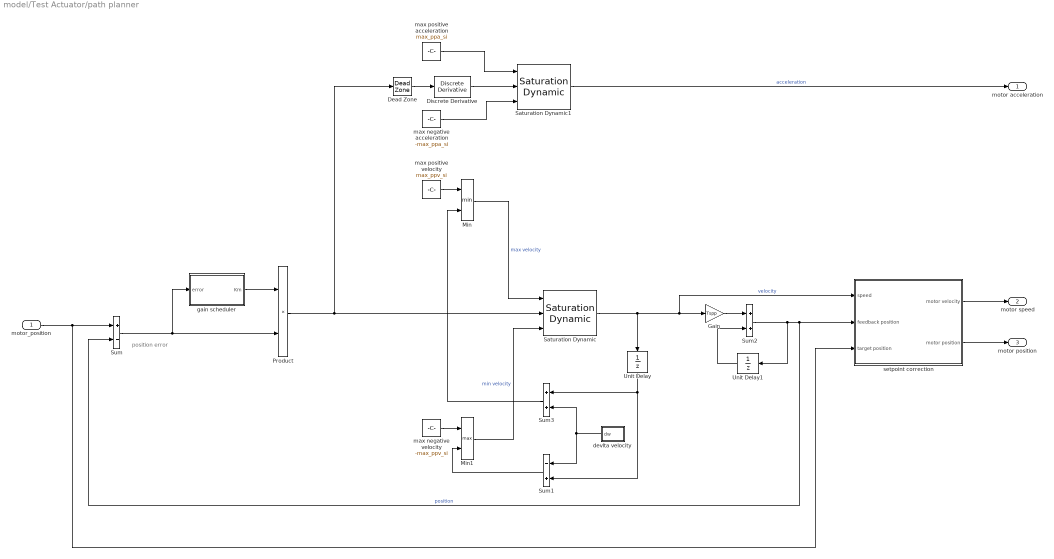
== system model/Test Actuator/path planner ==
  note: position error
  motor_position : Inport
  Dead Zone : DeadZone  LowerValue=-0.01  UpperValue=0.01
  Discrete Derivative : simulink/Discrete/Discrete Derivative  gainval=1.0  ICPrevScaledInput=0.0  OutMin=[]  OutMax=[]  OutDataType=fixdt(1, 16)  OutScaling=2^-10  DoSatur=off
  Gain : Gain  Gain=Tspp
  Min : MinMax  Inputs=2
  Min1 : MinMax  Function=max  Inputs=2
  Product : Product
  Saturation Dynamic : simulink/Discontinuities/Saturation Dynamic  OutMin=[]  OutMax=[]  OutDataTypeStr=Inherit: Same as second input  OutDataType=fixdt(1, 16)  OutScaling=2^-10  DoSatur=off
  Saturation Dynamic1 : simulink/Discontinuities/Saturation Dynamic  OutMin=[]  OutMax=[]  OutDataTypeStr=Inherit: Same as second input  OutDataType=fixdt(1, 16)  OutScaling=2^-10  DoSatur=off
  Sum : Sum  Inputs=+-
  Sum1 : Sum  Inputs=-+
  Sum2 : Sum
  Sum3 : Sum
  Unit Delay : UnitDelay  SampleTime=-1  HasFrameUpgradeWarning=on
  Unit Delay1 : UnitDelay  SampleTime=-1  HasFrameUpgradeWarning=on
  devlta velocity : Subsystem
  gain scheduler : Subsystem
  max negative acceleration : Constant  Value=-max_ppa_si
  max negative velocity : Constant  Value=-max_ppv_si
  max positive acceleration : Constant  Value=max_ppa_si
  max positive velocity : Constant  Value=max_ppv_si
  setpoint correction : Subsystem
  motor acceleration : Outport
  motor speed : Outport  Port=2
  motor position : Outport  Port=3
  wires:
  Sum/1 -> gain scheduler/1(error), Product/2
  max positive velocity/1 -> Min/1
  Saturation Dynamic/1 -> Gain/1, setpoint correction/1(speed), Unit Delay/1  "velocity"
  devlta velocity/1(dw) -> Sum1/1, Sum3/2
  Sum3/1 -> Min/2
  max negative velocity/1 -> Min1/1
  Sum1/1 -> Min1/2
  Min1/1 -> Saturation Dynamic/3  "min velocity"
  Min/1 -> Saturation Dynamic/1  "max velocity"
  Sum2/1 -> setpoint correction/2(feedback position), Sum/2, Unit Delay1/1  "position"
  Unit Delay/1 -> Sum3/1, Sum1/2
  max positive acceleration/1 -> Saturation Dynamic1/1
  max negative acceleration/1 -> Saturation Dynamic1/3
  Saturation Dynamic1/1 -> motor acceleration/1  "acceleration"
  Discrete Derivative/1 -> Saturation Dynamic1/2
  Dead Zone/1 -> Discrete Derivative/1
  setpoint correction/1(motor velocity) -> motor speed/1
  gain scheduler/1(Km) -> Product/1
  motor_position/1 -> setpoint correction/3(target position), Sum/1
  setpoint correction/2(motor position) -> motor position/1
  Product/1 -> Dead Zone/1, Saturation Dynamic/2
  Gain/1 -> Sum2/1
  Unit Delay1/1 -> Sum2/2

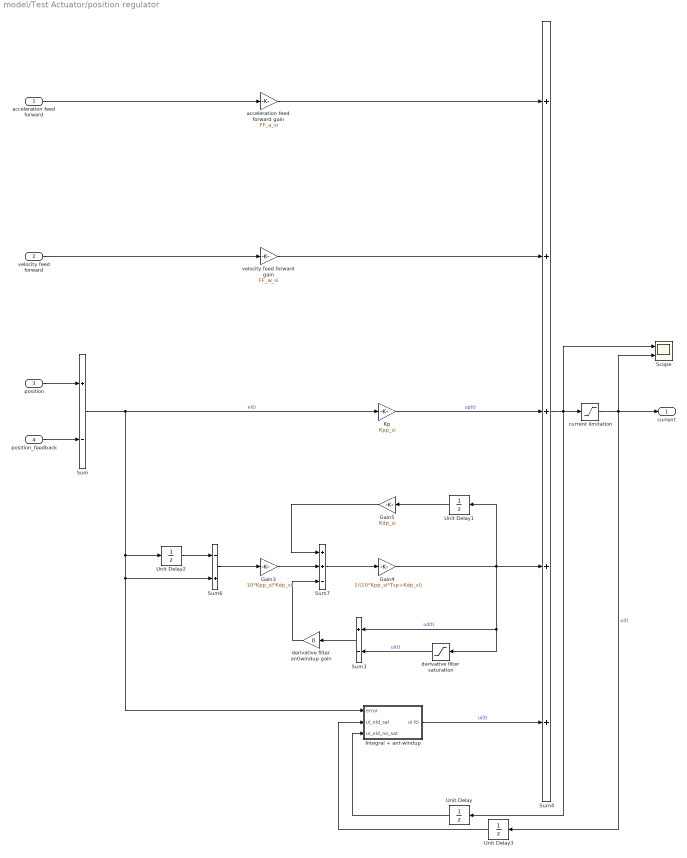
== system model/Test Actuator/position regulator ==
  acceleration feed forward : Inport
  velocity feed forward : Inport  Port=2
  position : Inport  Port=3
  position_feedback : Inport  Port=4
  Gain3 : Gain  Gain=10*Kpp_si*Kdp_si
  Gain4 : Gain  Gain=1/(10*Kpp_si*Tsp+Kdp_si)
  Gain5 : Gain  Gain=Kdp_si
  Integral + ant-windup : Subsystem
  Kp : Gain  Gain=Kpp_si
  Scope : Scope  NumInputPorts=2
  Sum : Sum  Inputs=+-
  Sum3 : Sum  Inputs=+-
  Sum4 : Sum  Inputs=+++++
  Sum6 : Sum  Inputs=-+
  Sum7 : Sum  Inputs=++-
  Unit Delay{,1..3} (4 alike) : UnitDelay  SampleTime=-1  HasFrameUpgradeWarning=on
  acceleration feed forward gain : Gain  Gain=FF_a_si
  current limitation : Saturate  UpperLimit=Imax  LowerLimit=-Imax
  derivative filter antiwindup gain : Gain  Gain=0
  derivative filter saturation : Saturate  UpperLimit=Imax/2  LowerLimit=-Imax/2
  velocity feed forward gain : Gain  Gain=FF_w_si
  current : Outport
  wires:
  acceleration feed forward gain/1 -> Sum4/1
  acceleration feed forward/1 -> acceleration feed forward gain/1
  velocity feed forward gain/1 -> Sum4/2
  velocity feed forward/1 -> velocity feed forward gain/1
  Sum7/1 -> Gain4/1
  current limitation/1 -> current/1, Scope/2, Unit Delay3/1  "u(t)"
  Unit Delay2/1 -> Sum6/1
  Sum6/1 -> Gain3/1
  Unit Delay1/1 -> Gain5/1
  Kp/1 -> Sum4/3  "up(t)"
  Sum/1 -> Kp/1, Integral + ant-windup/1(error), Sum6/2, Unit Delay2/1  "e(t)"
  Gain3/1 -> Sum7/2
  Gain5/1 -> Sum7/1
  Gain4/1 -> Sum4/4, derivative filter saturation/1, Sum3/1, Unit Delay1/1  "ud(t)"
  Sum3/1 -> derivative filter antiwindup gain/1
  derivative filter saturation/1 -> Sum3/2  "ui(t)"
  derivative filter antiwindup gain/1 -> Sum7/3
  Integral + ant-windup/1(ui (t)) -> Sum4/5  "ui(t)"
  Sum4/1 -> Scope/1, current limitation/1, Unit Delay/1
  position/1 -> Sum/1
  position_feedback/1 -> Sum/2
  Unit Delay/1 -> Integral + ant-windup/3(ui_old_no_sat)
  Unit Delay3/1 -> Integral + ant-windup/2(ui_old_sat)
